simulink model "AmpelkreuzungV2_5"  (R2024b)
settings: Solver=FixedStepAuto  StartTime=0.0  StopTime=100000  FixedStep=1  RelTol=1e-3
model workspace (MATLAB code in the model file):
  | function [autos_l1, autos_rg1, autos_2l, autos_2rg, autos_3l, autos_3rg, autos_4, fehler] = generateCars(Auslastung)
  |     if (auslastung == 1)
  |         autos_l1 = round(randn());
  |         autos_rg1 = round(randn());
  |         autos_2l = round(randn());
  |         autos_2rg = round(randn());
  |         autos_3l = round(randn());
  |         autos_3rg = round(randn());
  |         autos_4 = round(randn());
  |     else
  |         fehler = 1;
  |     end
  | 
  |     if (auslastung == 2)
  |         autos_l1 = round(randn());
  |         autos_rg1 = round(4 + 2 * randn());
  |         autos_2l = round(1 + randn());
  |         autos_2rg = round(4 + 2 * randn());
  |         autos_3l = round(randn());
  |         autos_3rg = round(2 + randn());
  |         autos_4 = round(1 + randn());
  |     else
  |         fehler = 1;
  |     end
  | 
  |     if (auslastung == 3)
  |         autos_l1 = round(1.5 + randn());
  |         autos_rg1 = round(7 + 2 * randn());
  |         autos_2l = round(2 + randn());
  |         autos_2rg = round(7 + 2 * randn());
  |         autos_3l = round(2 * randn());
  |         autos_3rg = round(3 + randn());
  |         autos_4 = round(2 + randn());
  |     else
  |         fehler = 1;
  |     end
  | 
  |     if (auslastung == 4)
  |         autos_l1 = round(2.5 + randn());
  |         autos_rg1 = round(13 + 3 * randn());
  |         autos_2l = round(5 + randn());
  |         autos_2rg = round(13 + 3 * randn());
  |         autos_3l = round(2 + randn());
  |         autos_3rg = round(2 + randn());
  |         autos_4 = round(5 + randn());
  |     else
  |         fehler = 1;
  |     end
  | end
settings Model: PacingRate=1000  Creator=richa  LastModifiedBy=lenna

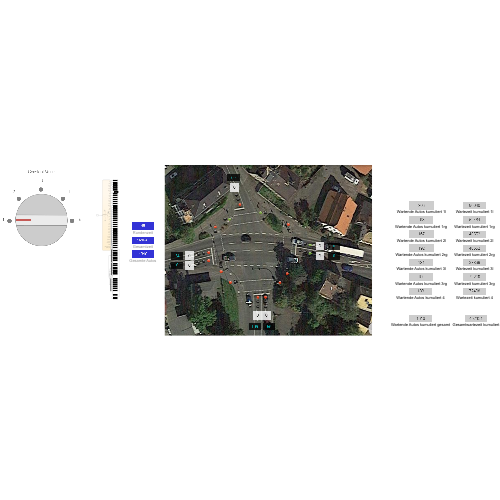
[thumbnail: Simulink's stored preview of the top-level diagram]
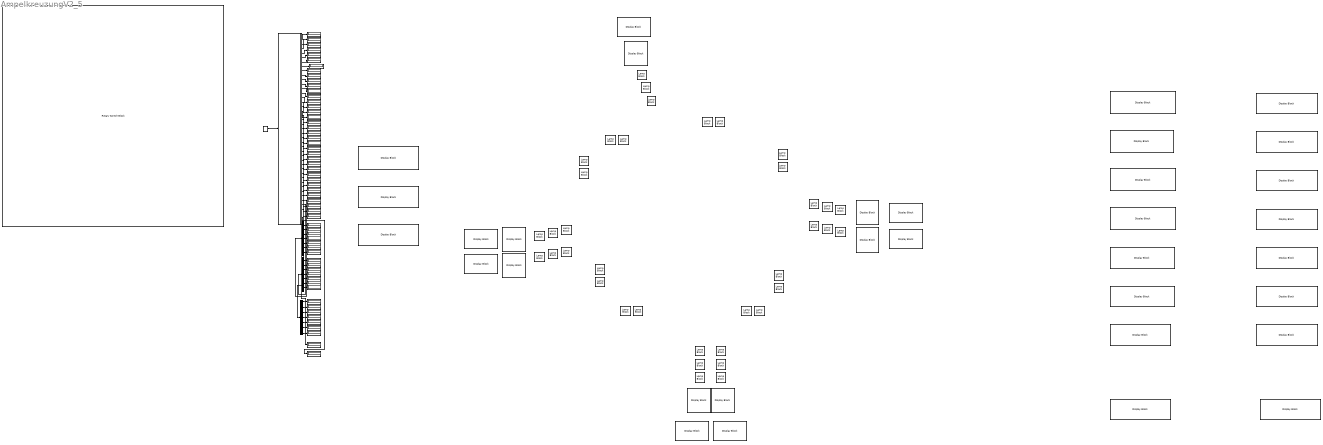
== system AmpelkreuzungV2_5 ==
  Chart : Stateflow chart  TreatAsAtomicUnit=on
  Constant : Constant
  Demux : Demux  Outputs=7
  Demux1 : Demux  Outputs=7
  Demux2 : Demux  Outputs=7
  Display{,1..26,28..33,38,41..44,46..51,58..70,76..77} (59 alike) : Display
  Display{27,34..37,39..40} (7 alike) : DisplayBlock  LabelPosition=Hide  Transparency=1  Layout=Fill available space
  Display{52..57,78} (7 alike) : DisplayBlock  LabelPosition=Hide  Transparency=1
  Gesamte Autos : DisplayBlock  LabelPosition=Hide  Transparency=1
  Gesamtwartezeit kumuliert : DisplayBlock  LabelPosition=Hide  Transparency=1
  Gesamtzeit : DisplayBlock  LabelPosition=Hide  Transparency=1
  Lamp{,1..36} (37 alike) : LampBlock  LabelPosition=Hide
  Rotary Switch : RotarySwitchBlock
      settings: Values={{'1', '2', '3', '4', '5'}, [1 2 3 4 5]}
  Rundenzeit : DisplayBlock  LabelPosition=Hide  Transparency=1
  Wartende Autos kumuliert 1l : DisplayBlock  LabelPosition=Hide  Transparency=1
  Wartende Autos kumuliert 1rg : DisplayBlock  LabelPosition=Hide  Transparency=1
  Wartende Autos kumuliert 2l : DisplayBlock  LabelPosition=Hide  Transparency=1
  Wartende Autos kumuliert 2rg : DisplayBlock  LabelPosition=Hide  Transparency=1
  Wartende Autos kumuliert 3l : DisplayBlock  LabelPosition=Hide  Transparency=1
  Wartende Autos kumuliert 3rg : DisplayBlock  LabelPosition=Hide  Transparency=1
  Wartende Autos kumuliert 4 : DisplayBlock  LabelPosition=Hide  Transparency=1
  Wartende Autos kumuliert gesamt : DisplayBlock  LabelPosition=Hide  Transparency=1
  Wartezeit kumuliert 1l : DisplayBlock  LabelPosition=Hide  Transparency=1
  Wartezeit kumuliert 1rg : DisplayBlock  LabelPosition=Hide  Transparency=1
  Wartezeit kumuliert 2l : DisplayBlock  LabelPosition=Hide  Transparency=1
  Wartezeit kumuliert 2rg : DisplayBlock  LabelPosition=Hide  Transparency=1
  Wartezeit kumuliert 3l : DisplayBlock  LabelPosition=Hide  Transparency=1
  Wartezeit kumuliert 3rg : DisplayBlock  LabelPosition=Hide  Transparency=1
  Wartezeit kumuliert 4 : DisplayBlock  LabelPosition=Hide  Transparency=1
  wires:
  Chart/1(rot1_l) -> Display/1
  Chart/2(gelb1_l) -> Display1/1
  Chart/3(gruen1_l) -> Display2/1
  Chart/4(rot1_rg) -> Display3/1
  Chart/5(gelb1_rg) -> Display4/1
  Chart/6(gruen1_rg) -> Display5/1
  Chart/7(rot2) -> Display6/1
  Chart/8(gelb2) -> Display7/1
  Chart/9(gruen2) -> Display8/1
  Chart/10(rot3_l) -> Display9/1
  Chart/11(gelb3_l) -> Display10/1
  Chart/12(gruen3_l) -> Display11/1
  Chart/13(rot3_rg) -> Display12/1
  Chart/14(gelb3_rg) -> Display13/1
  Chart/15(gruen3_rg) -> Display14/1
  Chart/16(rot4) -> Display15/1
  Chart/17(gelb4) -> Display16/1
  Chart/18(gruen4) -> Display17/1
  Chart/19(rot5) -> Display18/1
  Chart/20(gruen5) -> Display19/1
  Chart/21(rot6) -> Display20/1
  Chart/22(gruen6) -> Display21/1
  Chart/23(rot7) -> Display22/1
  Chart/24(gruen7) -> Display23/1
  Chart/25(rot8) -> Display24/1
  Chart/26(gruen8) -> Display25/1
  Chart/27(autos_1l) -> Display26/1
  Chart/28(autos_1rg) -> Display28/1
  Chart/29(autos_2l) -> Display29/1
  Chart/30(autos_2rg) -> Display30/1
  Chart/31(autos_3l) -> Display31/1
  Chart/32(autos_3rg) -> Display32/1
  Chart/33(autos_4) -> Display33/1
  Constant/1 -> Chart/1(auslastung_eingang)
  Chart/34(timeCounter) -> Display38/1
  Chart/35(gesamtZeit) -> Display42/1
  Chart/36(gesamteAutos) -> Display44/1
  Chart/37(timer_spuren) -> Demux/1
  Demux/1 -> Display46/1
  Demux/2 -> Display47/1
  Demux/3 -> Display48/1
  Demux/4 -> Display49/1
  Demux/5 -> Display50/1
  Demux/6 -> Display51/1
  Chart/38(wartende_autos) -> Demux1/1
  Chart/39(wartezeit) -> Demux2/1
  Demux1/1 -> Display58/1
  Demux1/2 -> Display59/1
  Demux1/3 -> Display60/1
  Demux1/4 -> Display61/1
  Demux1/5 -> Display62/1
  Demux1/6 -> Display63/1
  Demux1/7 -> Display64/1
  Demux2/1 -> Display65/1
  Demux2/2 -> Display66/1
  Demux2/3 -> Display67/1
  Demux2/4 -> Display68/1
  Demux2/5 -> Display69/1
  Demux2/6 -> Display70/1
  Demux/7 -> Display76/1
  Demux2/7 -> Display77/1
  Chart/40(gesamte_wartende_autos) -> Display43/1
  Chart/41(gesamte_wartezeit) -> Display41/1

== stateflow chart AmpelkreuzungV2_5/Chart ==
  state Start
    entry:
    rot1_l = 1;
    gelb1_l = 0;
    gruen1_l = 0;
    rot1_rg = 1;
    gelb1_rg = 0;
    gruen1_rg = 0;
    rot2 = 1;
    gelb2 = 0;
    gruen2 = 0;
    rot3_l = 1;
    gelb3_l = 0;
    gruen3_l = 0;
    rot3_rg = 1;
    gelb3_rg = 0;
    gruen3_rg = 0;
    rot4 = 1;
    gelb4 = 0;
    gruen4 = 0;
    rot5 = 1;
    gruen5 = 0;
    rot6 = 1;
    gruen6 = 0;
    rot7 = 1;
    gruen7 = 0;
    rot8 = 1;
    gruen8 = 0;
    restliche_autos = [0 0 0 0 0 0 0];
    timeCounter = 0;
    timer_spuren = [0 0 0 0 0 0 0];
    gesamtZeit = 0;
    gesamteAutos = 0;
    gekreuzteAutos = [0 0 0 0 0 0 0];
    wartende_autos = [0 0 0 0 0 0 0];
    wartezeit = [0 0 0 0 0 0 0];
    gesamte_wartende_autos = 0;
    gesamte_wartezeit = 0;
  state Autozuweisung
    entry:
    autos_1l = autos(1) + restliche_autos(1);
    autos_1rg = autos(2) + restliche_autos(2);
    autos_2l = autos(3) + restliche_autos(3);
    autos_2rg = autos(4) + restliche_autos(4);
    autos_3l = autos(5) + restliche_autos(5);
    autos_3rg = autos(6) + restliche_autos(6);
    autos_4 = autos(7) + restliche_autos(7);
  state runden_wartende_autos
    entry:
    runden_wartende_autos = [autos_1l, autos_1rg, autos_2l, autos_2rg, autos_3l, autos_3rg, autos_4]
  state l1_rg1_rotgelb
    entry:
    gelb1_l = 1;
    gelb1_rg = 1;
  state rg1_ampel2_rotgelb
    entry:
    gelb1_rg = 1;
    gelb2 = 1;
  state l1_rg1_gruen
    entry:
    rot1_l = 0;
    gelb1_l = 0;
    gruen1_l = 1;
    rot1_rg = 0;
    gelb1_rg = 0;
    gruen1_rg = 1;
    rot7 = 0;
    gruen7 = 1;
  state rg1_ampel2_gruen
    entry:
    rot1_rg = 0;
    gelb1_rg = 0;
    gruen1_rg = 1;
    rot2 = 0;
    gelb2 = 0;
    gruen2 = 1;
    rot7 = 0;
    gruen7 = 1;
    rot8 = 0;
    gruen8 = 1;
  state l1_gelb
    entry:
    gelb1_l = 1;
    gruen1_l = 0;
  state l1_rot
    entry:
    rot1_l = 1;
    gelb1_l = 0;
  state neu_autos1l
    entry:
    autos_1l = restliche_autos(1)
  state ampel2_rotgelb
    entry:
    gelb2 = 1;
  state Fuss7_rot1
    entry:
    rot7 = 1;
    gruen7 = 0;
  state ampel2_fuss8_gruen
    rot2 = 0;
    gelb2 = 0;
    gruen2 = 1;
    rot8 = 0;
    gruen8 = 1;
  state rg1_gelb1
    entry:
    gelb1_rg = 1;
    gruen1_rg = 0;
  state Fuss7_rot
    entry:
    rot7 = 1;
    gruen7 = 0;
  state rg1_gelb
    entry:
    gelb1_rg = 1;
    gruen1_rg = 0;
  state rg1_rot
    entry:
    gelb1_rg = 0;
    rot1_rg = 1;
  state neu_autos1rg2
    entry:
    autos_1rg = restliche_autos(2)
  state neu_autos1rg
    entry:
    autos_1rg = restliche_autos(2)
  state fuss8_rot1
    entry:
    rot8 = 1;
    gruen8 = 0;
  state fuss8_rot
    entry:
    rot8 = 1;
    gruen8 = 0;
  state ampel2_gelb1
    entry:
    gelb2 = 1;
    gruen2 = 0;
  state ampel2_gelb
    entry:
    gelb2 = 1;
    gruen2 = 0;
  state ampel2_rot1
    rot2 = 1;
    gelb2 = 0;
  state ampel2_rot
    rot2 = 1;
    gelb2 = 0;
  state neu_autos2l1
    entry:
    autos_2l = restliche_autos(3)
  state neu_autos2l
    entry:
    autos_2l = restliche_autos(3)
  state neu_autos2rg1
    entry:
    autos_2rg = restliche_autos(4)
  state neu_autos2rg
    entry:
    autos_2rg = restliche_autos(4)
  state rg3_rotgelb
    entry:
    gelb3_rg = 1;
  state rg3_rotgelb1
    entry:
    gelb3_rg = 1;
  state l3_rotgelb_rg3_fuss6_gruen
    entry:
    gelb3_l = 1;
    rot3_rg = 0;
    gelb3_rg = 0;
    gruen3_rg = 1;
    rot6 = 0;
    gruen6 = 1;
  state rg3_fuss6_gruen
    entry:
    rot3_rg = 0;
    gelb3_rg = 0;
    gruen3_rg = 1;
    rot6 = 0;
    gruen6 = 1;
  state l3_gruen
    entry:
    rot3_l = 0;
    gelb3_l = 0;
    gruen3_l = 1;
  state ampel4_rotgelb
    entry:
    gelb4 = 1;
  state l3_gelb
    entry:
    gelb3_l = 1;
    gruen3_l = 0;
  state ampel4_fuss5_gruen
    entry:
    rot4 = 0;
    gelb4 = 0;
    gruen4 = 1;
    rot5 = 0;
    gruen5 = 1;
  state l3_fuss6_rot
    entry:
    rot3_l = 1;
    gelb3_l = 0;
    rot6 = 1;
    gruen6 = 0;
  state fuss6_rot
    entry:
    rot6 = 1;
    gruen6 = 0;
  state neu_autos3l
    entry:
    autos_3l = restliche_autos(5)
  state rg3_gelb
    entry:
    gelb3_rg = 1;
    gruen3_rg = 0;
  state rg3_gelb1
    entry:
    gelb3_rg = 1;
    gruen3_rg = 0;
  state rg3_rot_ampel4_rotgelb
    entry:
    rot3_rg = 1;
    gelb3_rg = 0;
    gelb4 = 1;
  state rg3_fuss5_rot
    entry:
    rot3_rg = 1;
    gelb3_rg = 0;
    rot5 = 1;
    gruen5 = 0;
  state neu_autos3rg
    entry:
    autos_3rg = restliche_autos(6)
  state neu_autos3rg1
    entry:
    autos_3rg = restliche_autos(6)
  state ampel4_fuss5_gruen1
    entry:
    rot4 = 0;
    gelb4 = 0;
    gruen4 = 1;
    rot5 = 0;
    gruen5 = 1;
  state fuss5_rot
    entry:
    rot5 = 1;
    gruen5 = 0;
  state ampel4_gelb
    entry:
    gelb4 = 1;
    gruen4 = 0;
  state ampel4_rot
    entry:
    rot4 = 1;
    gelb4 = 0;
  state neu_autos4
    entry:
    autos_4 = restliche_autos(7)
  (default) -> Start
  Start -> (junction 248)
  (junction 181) -> (junction 248) : {timeCounter = resetTimer()}
  (junction 179) -> (junction 181)
  (junction 248) -> (junction 371) : {kapazitaet = generiereKapazitaet()}
  (junction 371) -> Autozuweisung : {autos = generiereAutos(auslastung_eingang)}
  Autozuweisung -> runden_wartende_autos
  runden_wartende_autos -> (junction 250)
  (junction 250) -> (junction 442) : after(1,sec)
      | {timeCounter = refresher(timeCounter, 1) }
  (junction 442) -> (junction 15) : {timer_spuren = countOnwards(timer_spuren,1,[1 1 1 1 1 1 1])}
      |
      | %Linksabbieger1
  (junction 15) -> (junction 69) [order 1] : [autos_1l == 0]
  (junction 15) -> (junction 17) [order 2]
  (junction 69) -> rg1_ampel2_rotgelb
  (junction 17) -> (junction 18) [order 1] : [autos_1l > 0]
  (junction 17) -> (junction 19) [order 2]
  (junction 18) -> l1_rg1_rotgelb
  l1_rg1_rotgelb -> (junction 444) : after(1,sec)
      | {timeCounter = refresher(timeCounter, 1) }
  (junction 444) -> (junction 468) : {timer_spuren = countOnwards(timer_spuren,1,[1 1 1 1 1 1 1])}
  (junction 468) -> l1_rg1_gruen : {[timer_spuren, wartende_autos, wartezeit, gesamte_wartende_autos, gesamte_wartezeit] = multifunction(timer_spuren,[1 1 0 0 0 0 0],wartezeit,runden_wartende_autos, wartende_autos, gesamte_wartende_autos, gesamte_wartezeit)}
  rg1_ampel2_rotgelb -> (junction 479) : after(1,sec)
      | {timeCounter = refresher(timeCounter, 1) }
  (junction 479) -> (junction 481) : {timer_spuren = countOnwards(timer_spuren,1,[1 1 1 1 1 1 1])}
  (junction 481) -> rg1_ampel2_gruen : {[timer_spuren, wartende_autos, wartezeit, gesamte_wartende_autos, gesamte_wartezeit] = multifunction(timer_spuren,[0 1 1 1 0 0 0],wartezeit,runden_wartende_autos,wartende_autos, gesamte_wartende_autos, gesamte_wartezeit)}
  l1_rg1_gruen -> (junction 446) : after(7,sec)
      | {timeCounter = refresher(timeCounter, 7) }
  (junction 446) -> l1_gelb : {timer_spuren = countOnwards(timer_spuren,7,[0 0 1 1 1 1 1])}
  l1_gelb -> (junction 449) : after(3,sec)
      | {timeCounter = refresher(timeCounter, 3) }
  rg1_ampel2_gruen -> (junction 483) : after(25,sec)
      | {timeCounter = refresher(timeCounter, 25) }
  (junction 449) -> l1_rot : {timer_spuren = countOnwards(timer_spuren,3,[0 0 1 1 1 1 1])}
  l1_rot -> (junction 407) : {restliche_autos(1) = subtrahiereAutos(autos_1l, kapazitaet(1))}
  (junction 407) -> neu_autos1l : {gesamteAutos = berechneGesamteAutos(gesamteAutos, autos(1), kapazitaet(1))}
  (junction 483) -> Fuss7_rot1 : {timer_spuren = countOnwards(timer_spuren,25,[1 0 0 0 1 1 1])}
  neu_autos1l -> (junction 451) : after(3,sec)
      | {timeCounter = refresher(timeCounter, 3) }
  (junction 451) -> ampel2_rotgelb : {timer_spuren = countOnwards(timer_spuren,3,[1 0 1 1 1 1 1])}
  ampel2_rotgelb -> (junction 464) : after(1,sec)
      | {timeCounter = refresher(timeCounter, 1) }
  (junction 464) -> (junction 466) : {timer_spuren = countOnwards(timer_spuren,1,[1 0 1 1 1 1 1])}
  (junction 466) -> ampel2_fuss8_gruen : {[timer_spuren, wartende_autos, wartezeit, gesamte_wartende_autos, gesamte_wartezeit] = multifunction(timer_spuren,[0 0 1 1 0 0 0],wartezeit, runden_wartende_autos,wartende_autos, gesamte_wartende_autos, gesamte_wartezeit)}
  Fuss7_rot1 -> (junction 485) : after(2,sec)
      | {timeCounter = refresher(timeCounter, 2) }
  ampel2_fuss8_gruen -> (junction 473) : after(25,sec)
      | {timeCounter = refresher(timeCounter, 25) }
  (junction 485) -> rg1_gelb1 : {timer_spuren = countOnwards(timer_spuren,2,[1 0 0 0 1 1 1])}
  (junction 473) -> Fuss7_rot : {timer_spuren = countOnwards(timer_spuren,25,[1 0 0 0 1 1 1])}
  rg1_gelb1 -> (junction 487) : after(3,sec)
      | {timeCounter = refresher(timeCounter, 3) }
  Fuss7_rot -> (junction 475) : after(2,sec)
      | {timeCounter = refresher(timeCounter, 2) }
  (junction 475) -> rg1_gelb : {timer_spuren = countOnwards(timer_spuren,2,[1 0 0 0 1 1 1])}
  (junction 487) -> (junction 71) : {timer_spuren = countOnwards(timer_spuren,3,[1 0 0 0 1 1 1])}
  rg1_gelb -> (junction 477) : after(3,sec)
      | {timeCounter = refresher(timeCounter, 3) }
  (junction 477) -> (junction 20) : {timer_spuren = countOnwards(timer_spuren,3,[1 0 0 0 1 1 1])}
  (junction 20) -> (junction 19)
  (junction 71) -> (junction 20)
  (junction 19) -> rg1_rot
  rg1_rot -> (junction 418) : {restliche_autos(2) = subtrahiereAutos(autos_1rg, kapazitaet(3))}
  (junction 418) -> (junction 199) : {gesamteAutos = berechneGesamteAutos(gesamteAutos, autos(2), kapazitaet(3))}
      |
      | %Linksabbieger2
  (junction 199) -> (junction 200) [order 1] : [autos_2l <= 2]
  (junction 199) -> (junction 201) [order 2]
  (junction 200) -> neu_autos1rg2
  (junction 201) -> (junction 202) [order 1] : [autos_2l > 2]
  (junction 201) -> (junction 203) [order 2]
  (junction 202) -> neu_autos1rg
  neu_autos1rg2 -> (junction 498) : after(7,sec)
      | {timeCounter = refresher(timeCounter, 7) }
  neu_autos1rg -> (junction 489) : after(20,sec)
      | {timeCounter = refresher(timeCounter, 20) }
  (junction 498) -> fuss8_rot1 : {timer_spuren = countOnwards(timer_spuren,7,[1 1 0 0 1 1 1])}
  (junction 489) -> fuss8_rot : {timer_spuren = countOnwards(timer_spuren,20,[1 1 0 0 1 1 1])}
  fuss8_rot1 -> (junction 500) : after(2,sec)
      | {timeCounter = refresher(timeCounter, 2) }
  fuss8_rot -> (junction 491) : after(2,sec)
      | {timeCounter = refresher(timeCounter, 2) }
  (junction 500) -> ampel2_gelb1 : {timer_spuren = countOnwards(timer_spuren,2,[1 1 0 0 1 1 1])}
  (junction 491) -> ampel2_gelb : {timer_spuren = countOnwards(timer_spuren,2,[1 1 0 0 1 1 1])}
  ampel2_gelb1 -> (junction 502) : after(3,sec)
      | {timeCounter = refresher(timeCounter, 3) }
  ampel2_gelb -> (junction 493) : after(3,sec)
      | {timeCounter = refresher(timeCounter, 3) }
  (junction 502) -> ampel2_rot1 : {timer_spuren = countOnwards(timer_spuren,3,[1 1 0 0 1 1 1])}
  (junction 493) -> ampel2_rot : {timer_spuren = countOnwards(timer_spuren,3,[1 1 0 0 1 1 1])}
  ampel2_rot1 -> (junction 423) : {restliche_autos(3) = subtrahiereAutos(autos_2l, kapazitaet(4))}
  ampel2_rot -> (junction 419) : {restliche_autos(3) = subtrahiereAutos(autos_2l, kapazitaet(5))}
  (junction 423) -> neu_autos2l1 : {gesamteAutos = berechneGesamteAutos(gesamteAutos, autos(3), kapazitaet(4))}
  (junction 419) -> neu_autos2l : {gesamteAutos = berechneGesamteAutos(gesamteAutos, autos(3), kapazitaet(5))}
  neu_autos2l1 -> (junction 426) : {restliche_autos(4) = subtrahiereAutos(autos_2rg, kapazitaet(6))}
  neu_autos2l -> (junction 421) : {restliche_autos(4) = subtrahiereAutos(autos_2rg, kapazitaet(7))}
  (junction 426) -> neu_autos2rg1 : {gesamteAutos = berechneGesamteAutos(gesamteAutos, autos(4), kapazitaet(6))}
  (junction 421) -> neu_autos2rg : {gesamteAutos = berechneGesamteAutos(gesamteAutos, autos(4), kapazitaet(7))}
  neu_autos2rg1 -> (junction 504) : after(1,sec)
      | {timeCounter = refresher(timeCounter, 1) }
  neu_autos2rg -> (junction 495) : after(1,sec)
      | {timeCounter = refresher(timeCounter, 1) }
  (junction 504) -> rg3_rotgelb1 : {timer_spuren = countOnwards(timer_spuren,1,[1 1 1 1 1 1 1])}
  (junction 495) -> rg3_rotgelb : {timer_spuren = countOnwards(timer_spuren,1,[1 1 1 1 1 1 1])}
  rg3_rotgelb -> (junction 204)
  rg3_rotgelb1 -> (junction 205)
  (junction 204) -> (junction 203)
  (junction 205) -> (junction 204)
  (junction 203) -> (junction 506) : {[timer_spuren, wartende_autos, wartezeit, gesamte_wartende_autos, gesamte_wartezeit] = multifunction(timer_spuren,[0 0 0 0 0 1 0],wartezeit,runden_wartende_autos,wartende_autos, gesamte_wartende_autos, gesamte_wartezeit)}
  (junction 506) -> (junction 115) : %Linksabbieger3
  (junction 115) -> (junction 116) [order 1] : [autos_3l == 0]
  (junction 116) -> (junction 526) : after(1,sec)
      | {timeCounter = refresher(timeCounter, 1) }
  (junction 115) -> (junction 117) [order 2]
  (junction 117) -> (junction 118) [order 1] : [autos_3l > 0]
  (junction 117) -> (junction 119) [order 2]
  (junction 118) -> l3_rotgelb_rg3_fuss6_gruen
  (junction 526) -> rg3_fuss6_gruen : {timer_spuren = countOnwards(timer_spuren,1,[1 1 1 1 1 1 1])}
  l3_rotgelb_rg3_fuss6_gruen -> (junction 508) : after(1,sec)
      | {timeCounter = refresher(timeCounter, 1) }
  (junction 508) -> (junction 510) : {timer_spuren = countOnwards(timer_spuren,1,[1 1 1 1 1 0 1])}
  rg3_fuss6_gruen -> (junction 530) : after(4,sec)
      | {timeCounter = refresher(timeCounter, 4) }
  (junction 510) -> l3_gruen : {[timer_spuren, wartende_autos, wartezeit, gesamte_wartende_autos, gesamte_wartezeit] = multifunction(timer_spuren,[0 0 0 0 1 0 0],wartezeit,runden_wartende_autos,wartende_autos, gesamte_wartende_autos, gesamte_wartezeit)}
  (junction 530) -> ampel4_rotgelb : {timer_spuren = countOnwards(timer_spuren,4,[1 1 1 1 1 0 1])}
  l3_gruen -> (junction 512) : after(8,sec)
      | {timeCounter = refresher(timeCounter, 8) }
  ampel4_rotgelb -> (junction 532) : after(1,sec)
      | {timeCounter = refresher(timeCounter, 1) }
  (junction 512) -> l3_gelb : {timer_spuren = countOnwards(timer_spuren,8,[1 1 1 1 0 0 1])}
  (junction 532) -> (junction 534) : {timer_spuren = countOnwards(timer_spuren,1,[1 1 1 1 1 0 1])}
  l3_gelb -> (junction 514) : after(3,sec)
      | {timeCounter = refresher(timeCounter, 3) }
  (junction 534) -> ampel4_fuss5_gruen : {[timer_spuren, wartende_autos, wartezeit, gesamte_wartende_autos, gesamte_wartezeit] = multifunction(timer_spuren,[0 0 0 0 0 0 1],wartezeit,runden_wartende_autos,wartende_autos, gesamte_wartende_autos, gesamte_wartezeit)}
  (junction 514) -> l3_fuss6_rot : {timer_spuren = countOnwards(timer_spuren,3,[1 1 1 1 0 0 1])}
  ampel4_fuss5_gruen -> (junction 536) : after(6,sec)
      | {timeCounter = refresher(timeCounter, 6) }
  l3_fuss6_rot -> (junction 428) : {restliche_autos(5) = subtrahiereAutos(autos_3l, kapazitaet(8))}
  (junction 536) -> fuss6_rot : {timer_spuren = countOnwards(timer_spuren,6,[1 1 1 1 1 0 0])}
  (junction 428) -> neu_autos3l : {gesamteAutos = berechneGesamteAutos(gesamteAutos, autos(5), kapazitaet(8))}
  fuss6_rot -> (junction 538) : after(2,sec)
      | {timeCounter = refresher(timeCounter, 2) }
  neu_autos3l -> (junction 516) : after(2,sec)
      | {timeCounter = refresher(timeCounter, 2) }
  (junction 538) -> rg3_gelb : {timer_spuren = countOnwards(timer_spuren,2,[1 1 1 1 1 0 0])}
  (junction 516) -> rg3_gelb1 : {timer_spuren = countOnwards(timer_spuren,2,[1 1 1 1 1 0 1])}
  rg3_gelb -> (junction 540) : after(3,sec)
      | {timeCounter = refresher(timeCounter, 3) }
  rg3_gelb1 -> (junction 518) : after(3,sec)
      | {timeCounter = refresher(timeCounter, 3) }
  (junction 540) -> rg3_fuss5_rot : {timer_spuren = countOnwards(timer_spuren,3,[1 1 1 1 1 0 0])}
  (junction 518) -> rg3_rot_ampel4_rotgelb : {timer_spuren = countOnwards(timer_spuren,3,[1 1 1 1 1 0 1])}
  rg3_rot_ampel4_rotgelb -> (junction 431) : {restliche_autos(6) = subtrahiereAutos(autos_3rg, kapazitaet(9))}
  rg3_fuss5_rot -> (junction 430) : {restliche_autos(6) = subtrahiereAutos(autos_3rg, kapazitaet(9))}
  (junction 431) -> neu_autos3rg : {gesamteAutos = berechneGesamteAutos(gesamteAutos, autos(6), kapazitaet(9))}
  (junction 430) -> neu_autos3rg1 : {gesamteAutos = berechneGesamteAutos(gesamteAutos, autos(6), kapazitaet(9))}
  neu_autos3rg -> (junction 520) : after(1,sec)
      | {timeCounter = refresher(timeCounter, 1) }
  neu_autos3rg1 -> (junction 121)
  (junction 520) -> (junction 522) : {timer_spuren = countOnwards(timer_spuren,1,[1 1 1 1 1 1 1])}
  (junction 522) -> ampel4_fuss5_gruen1 : {[timer_spuren, wartende_autos, wartezeit, gesamte_wartende_autos, gesamte_wartezeit] = multifunction(timer_spuren,[0 0 0 0 0 0 1],wartezeit,runden_wartende_autos,wartende_autos, gesamte_wartende_autos, gesamte_wartezeit)}
  ampel4_fuss5_gruen1 -> (junction 524) : after(11,sec)
      | {timeCounter = refresher(timeCounter, 11) }
  (junction 524) -> fuss5_rot : {timer_spuren = countOnwards(timer_spuren,11,[1 1 1 1 1 1 0])}
  fuss5_rot -> (junction 120)
  (junction 121) -> (junction 120)
  (junction 120) -> (junction 119)
  (junction 119) -> (junction 122) : after(2,sec)
      | {timeCounter = refresher(timeCounter, 2) }
  (junction 122) -> ampel4_gelb : {timer_spuren = countOnwards(timer_spuren,2,[1 1 1 1 1 1 0])}
  ampel4_gelb -> (junction 543) : after(3,sec)
      | {timeCounter = refresher(timeCounter, 3) }
  (junction 543) -> ampel4_rot : {timer_spuren = countOnwards(timer_spuren,3,[1 1 1 1 1 1 0])}
  ampel4_rot -> (junction 433) : {restliche_autos(7) = subtrahiereAutos(autos_4, kapazitaet(10))}
  (junction 433) -> neu_autos4 : {gesamteAutos = berechneGesamteAutos(gesamteAutos, autos(7), kapazitaet(10))}
  neu_autos4 -> (junction 545) : after(4,sec)
      | {timeCounter = refresher(timeCounter, 4) }
  (junction 545) -> (junction 395) : {timer_spuren = countOnwards(timer_spuren,4,[1 1 1 1 1 1 1])}
  (junction 395) -> (junction 177) : {gesamtZeit = gesamtZeit + timeCounter;}
  (junction 177) -> (junction 179)
  data: maximale_kapazitaet function_output; anzahl_autos_pro_spur function_output; auslastung function_input; time function_input; timeElapsed function_input; spuren function_input; count_spur function_output; timer function_input; spuren function_input; ges_gewartete_zeit function_input; resetted_time function_output; gewartete_autos function_input; ges_gewartete_autos function_input; ges_gewartete_autos function_output; ges_gewartete_zeit function_output; ges_wartende_autos function_input; ges_wartezeit function_input; ges_wartende_autos function_output; ges_wartezeit function_output; anzahl_autos_pro_spur function_input; verbleibende_autos function_output; maximale_kapazitaet function_input; timer function_output; timer function_output; startTime function_input; timeElapsed function_input; anzahlGesamterAutos function_input; autosX function_input; maxKapazitaet function_input; anzahlGesamterAutos function_output; rot1_l output; gelb1_l output; gruen1_l output; rot1_rg output; gelb1_rg output; gruen1_rg output; rot2 output; gelb2 output; gruen2 output; rot3_l output; gelb3_l output; gruen3_l output; rot3_rg output; gelb3_rg output; gruen3_rg output; rot4 output; gelb4 output; gruen4 output; rot5 output; gruen5 output; rot6 output; gruen6 output; rot7 output; gruen7 output; rot8 output; gruen8 output; autos_1l output; autos_1rg output; autos_2l output; autos_2rg output; autos_3l output; autos_3rg output; autos_4 output; autos local; auslastung_eingang input; restliche_autos local; kapazitaet local; timeCounter output; gesamtZeit output; gesamteAutos output; gekreuzteAutos local; timer_spuren output; wartende_autos output; wartezeit output; runden_wartende_autos local; gesamte_wartende_autos output; gesamte_wartezeit output
  function maximale_kapazitaet = generiereKapazitaet:
    | function maximale_kapazitaet = generiereKapazitaet()
    |     maximale_kapazitaet = [5 + randn(),  20 + 3 * randn(), 30 + 3 * randn(), 5 + 2 * randn(), 8 + 2 * randn(), 20 + 3 * randn(),  25 + 3 * randn(), 5 + randn(), 8 + 2 * randn(), 8 + 2 * randn()];
    |     untere_kapazitaet = [3, 15, 22, 3, 5, 15, 19, 3, 5, 5];
    |     obere_kapazitaet = [7, 25, 35, 7, 10, 25, 32, 7, 10, 10];
    |     for i = 1:10
    |         if maximale_kapazitaet(i) < untere_kapazitaet(i)
    |             maximale_kapazitaet(i) = round(untere_kapazitaet(i));
    |         elseif maximale_kapazitaet(i) > obere_kapazitaet(i)
    |             maximale_kapazitaet(i) = round(obere_kapazitaet(i));
    |         else
    |             maximale_kapazitaet(i) = round(maximale_kapazitaet(i));
    |         end
    |     end
    | end
  function anzahl_autos_pro_spur = generiereAutos(auslastung):
    | function anzahl_autos_pro_spur = generiereAutos(auslastung)
    | 
    |     if (auslastung == 1)
    |         autos_1l = round(0.5 * randn());
    |         autos_1rg = round(0.5 * randn());
    |         autos_2l = round(0.5 * randn());
    |         autos_2rg = round(0.5 * randn());
    |         autos_3l = round(0.5 * randn());
    |         autos_3rg = round(0.5 * randn());
    |         autos_4 = round(0.5 * randn());
    |     elseif (auslastung == 2)
    |         autos_1l = round(randn());
    |         autos_1rg = round(4 + 2 * randn());
    |         autos_2l = round(1 + randn());
    |         autos_2rg = round(4 + 2 * randn());
    |         autos_3l = round(randn());
    |         autos_3rg = round(2 + randn());
    |         autos_4 = round(1 + randn());
    |     elseif (auslastung == 3)
    |         autos_1l = round(1.5 + randn());
    |         autos_1rg = round(7 + 2 * randn());
    |         autos_2l = round(2 + randn());
    |         autos_2rg = round(7 + 2 * randn());
    |         autos_3l = round(2 * randn());
    |         autos_3rg = round(3 + randn());
    |         autos_4 = round(2 + randn());
    |     elseif (auslastung == 4)
    |         autos_1l = round(2.5 + randn());
    |         autos_1rg = round(13 + 3 * randn());
    |         autos_2l = round(5 + randn());
    |         autos_2rg = round(13 + 3 * randn());
    |         autos_3l = round(2 + randn());
    |         autos_3rg = round(5 + randn());
    |         autos_4 = round(5 + randn());
    |     elseif (auslastung == 5)
    |         autos_1l = round(3.5 + randn());
    |         autos_1rg = round(20 + 5 * randn());
    |         autos_2l = round(7 + 2* randn());
    |         autos_2rg = round(20 + 5 * randn());
    |         autos_3l = round(5 + 2 * randn());
    |         autos_3rg = round(8 + 2 * randn());
    |         autos_4 = round(8 + 2 * randn());
    |     else
    |         autos_1l = 0;
    |         autos_1rg = 0;
    |         autos_2l = 0;
    |         autos_2rg = 0;
    |         autos_3l = 0;
    |         autos_3rg = 0;
    |         autos_4 = 0;
    |     end
    | 
    |     anzahl_autos_pro_spur = [autos_1l, autos_1rg, autos_2l, autos_2rg, autos_3l, autos_3rg, autos_4];
    | 
    |     for i = 1:(length(anzahl_autos_pro_spur))
    |         if anzahl_autos_pro_spur(i) < 0
    |             anzahl_autos_pro_spur(i) = 0;
    |         end
    |     end
    | end
  function count_spur = countOnwards(time, timeElapsed, spuren):
    | function count_spur = countOnwards(time, timeElapsed, spuren)
    |     count_spur = time;
    |     i = 1;
    |     for i = 1 : length(time)
    |         if spuren(i) == 1
    |             count_spur(i) = count_spur(i) + timeElapsed;
    |         end
    |     end
    | end
  function [resetted_time, ges_gewartete_autos, ges_gewartete_zeit, ges_wartende_autos, ges_wartezeit] = multifunction(timer,spuren,ges_gewartete_zeit, gewartete_autos, ges_gewartete_autos, ges_wartende_autos, ges_wartezeit):
    | function [resetted_time, ges_gewartete_autos, ges_gewartete_zeit, ges_wartende_autos, ges_wartezeit] = multifunction(timer,spuren,ges_gewartete_zeit, gewartete_autos, ges_gewartete_autos, ges_wartende_autos, ges_wartezeit)
    |     resetted_time = timer;
    |     for i = 1 : length(spuren)
    |         if spuren(i) == 1
    |             resetted_time(i) = 0;
    |             ges_gewartete_autos(i) = ges_gewartete_autos(i) + gewartete_autos(i);
    |             ges_gewartete_zeit(i) = ges_gewartete_zeit(i) + timer(i);
    |             ges_wartende_autos = ges_wartende_autos + gewartete_autos(i);
    |             ges_wartezeit = ges_wartezeit + timer(i);
    |         end
    |     end
    | end
  function verbleibende_autos = subtrahiereAutos(anzahl_autos_pro_spur, maximale_kapazitaet):
    | function verbleibende_autos = subtrahiereAutos(anzahl_autos_pro_spur, maximale_kapazitaet)
    |     verbleibende_autos = round(anzahl_autos_pro_spur - maximale_kapazitaet);
    |     if (verbleibende_autos < 0)
    |         verbleibende_autos = 0;
    |     end
    | end
  function timer = resetTimer:
    | function timer = resetTimer()
    |     timer = 0;
    | end
  function timer = refresher(startTime, timeElapsed):
    | function timer = refresher(startTime, timeElapsed)
    |     timer = startTime + timeElapsed;
    | end
  function anzahlGesamterAutos = berechneGesamteAutos(anzahlGesamterAutos, autosX, maxKapazitaet):
    | function anzahlGesamterAutos = berechneGesamteAutos(anzahlGesamterAutos, autosX, maxKapazitaet)
    |     if autosX > maxKapazitaet
    |         anzahlGesamterAutos = anzahlGesamterAutos + maxKapazitaet;
    |     else
    |         anzahlGesamterAutos = anzahlGesamterAutos + autosX;
    |     end
    | end
